simulink model "Pokus09_Display_4x4"  (Simulink 8.1)
settings: Solver=FixedStepDiscrete  StartTime=0.0  StopTime=10.0  RelTol=1e-3
libraries: simulink_extras x1, Displays_Lib x1, Computer_Library x1
settings Model: Creator=uzivatel  LastModifiedBy=uzivatel  SimulationMode=accelerator
settings DataIOCC: SignalLoggingSaveFormat=Dataset
settings OptimizationCC: ExpressionDepthLimit=128
settings DebuggingCC: FcnCallInpInsideContextMsg=EnableAllAsError
settings ModelReferenceCC: UpdateModelReferenceTargets=AssumeUpToDate  CheckModelReferenceTargetMessage=none
settings GRTTargetCC: CombineOutputUpdateFcns=on  GRTInterface=off

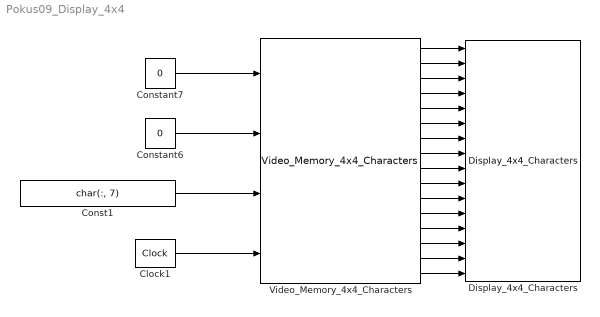
== system Pokus09_Display_4x4 ==
  Clock1 : simulink_extras/Flip Flops/Clock  period=1
  Const1 : Constant  Value=char(:, 7)  OutDataTypeStr=uint8
  Constant6 : Constant  Value=0  OutDataTypeStr=uint8
  Constant7 : Constant  Value=0  OutDataTypeStr=uint8
  Display_4x4_Characters : Displays_Lib/Displays_Lib/Display_4x4_Characters
  Video_Memory_4x4_Characters : Computer_Library/Video_Memory_4x4_Characters
  wires:
  Video_Memory_4x4_Characters/1 -> Display_4x4_Characters/1
  Video_Memory_4x4_Characters/2 -> Display_4x4_Characters/2
  Video_Memory_4x4_Characters/3 -> Display_4x4_Characters/3
  Video_Memory_4x4_Characters/4 -> Display_4x4_Characters/4
  Video_Memory_4x4_Characters/5 -> Display_4x4_Characters/5
  Video_Memory_4x4_Characters/6 -> Display_4x4_Characters/6
  Video_Memory_4x4_Characters/7 -> Display_4x4_Characters/7
  Video_Memory_4x4_Characters/8 -> Display_4x4_Characters/8
  Video_Memory_4x4_Characters/9 -> Display_4x4_Characters/9
  Video_Memory_4x4_Characters/10 -> Display_4x4_Characters/10
  Video_Memory_4x4_Characters/11 -> Display_4x4_Characters/11
  Video_Memory_4x4_Characters/12 -> Display_4x4_Characters/12
  Video_Memory_4x4_Characters/13 -> Display_4x4_Characters/13
  Video_Memory_4x4_Characters/14 -> Display_4x4_Characters/14
  Video_Memory_4x4_Characters/15 -> Display_4x4_Characters/15
  Video_Memory_4x4_Characters/16 -> Display_4x4_Characters/16
  Constant7/1 -> Video_Memory_4x4_Characters/1
  Constant6/1 -> Video_Memory_4x4_Characters/2
  Const1/1 -> Video_Memory_4x4_Characters/3
  Clock1/1 -> Video_Memory_4x4_Characters/4
